simulink model "kopter_se_zavazim_Cascade_PID"  (R2024b)
settings: Solver=ode4  StartTime=0.0  StopTime=16  FixedStep=0.01  RelTol=1e-3
values from neighbouring files (symbols this model uses):
  A = 0.6081    [parametry_kopter_se_zavazim.m]
  b_moment = 3.6e-7    (= 3.6e-07)    [parametry_kopter_se_zavazim.m]
  d = 1    [parametry_kopter_se_zavazim.m]
  g = 9.81    [parametry_kopter_se_zavazim.m]
  Ip = m*d^2    (= 1)    [parametry_kopter_se_zavazim.m]
  Ixx = 0.0222    [parametry_kopter_se_zavazim.m]
  Iyy = 0.0222    [parametry_kopter_se_zavazim.m]
  Izz = 0.0429    [parametry_kopter_se_zavazim.m]
  k_thrust = 9.3e-6    (= 9.3e-06)    [parametry_kopter_se_zavazim.m]
  l = 0.2051    [parametry_kopter_se_zavazim.m]
  M = 2    [parametry_kopter_se_zavazim.m]
  m = 1    [parametry_kopter_se_zavazim.m]
  T = 0.8682    [parametry_kopter_se_zavazim.m]
  Us = [(M+m)*g; 0; 0; 0]    [parametry_kopter_se_zavazim.m]
  Xinit_ss = [Xinit_matrix; [0 0 0 0 0 0 0 0]']    [parametry_kopter_se_zavazim.m]
  Xs = [0;0;0; 0;0;0; 0;0; 0;0;0; 0;0;0; 0;0]    [parametry_kopter_se_zavazim.m]
undefined symbols (not defined in the file or in its folder): L, Us_p, Xs_p
libraries: simulink_extras x21, slpidlib x21, simulink x6
(part 5 of 5)

== matlab function kopter_se_zavazim_Cascade_PID/Nelinearni State-Space/B ==
  data: roll input; B output; pitch input; yaw input; alpha input; beta input; M parameter; Ixx parameter; Iyy parameter; Izz parameter; Ip parameter; d parameter; m parameter
function B = fcn(roll, pitch, yaw, alpha, beta, M, Ixx, Iyy, Izz, Ip, d, m)
% Matice vstupu do soustavy kvadrokoptery se zavazim

phi_t = roll;
theta_t = pitch;
psi_t = yaw;

alpha_t = alpha;
beta_t = beta;

B = [ 
                                                                                                                                                                                                                                                                                                                                                                                                                                                                                                                                                                                   0,                                                                                                                                                                           0,                                                                        0,                                                                                          0;
                                                                                                                                                                                                                                                                                                                                                                                                                                                                                                                                                                                   0,                                                                                                                                                                           0,                                                                        0,                                                                                          0;
                                                                                                                                                                                                                                                                                                                                                                                                                                                                                                                                                                                   0,                                                                                                                                                                           0,                                                                        0,                                                                                          0;
                                                                                                                                                                                                                                                                                                                                                                                                                                                                                                                                                                                   0,                                                                                                                                                                           0,                                                                        0,                                                                                          0;
                                                                                                                                                                                                                                                                                                                                                                                                                                                                                                                                                                                   0,                                                                                                                                                                           0,                                                                        0,                                                                                          0;
                                                                                                                                                                                                                                                                                                                                                                                                                                                                                                                                                                                   0,                                                                                                                                                                           0,                                                                        0,                                                                                          0;
                                                                                                                                                                                                                                                                                                                                                                                                                                                                                                                                                                                   0,                                                                                                                                                                           0,                                                                        0,                                                                                          0;
                                                                                                                                                                                                                                                                                                                                                                                                                                                                                                                                                                                   0,                                                                                                                                                                           0,                                                                        0,                                                                                          0;
(M*sin(phi_t)*sin(psi_t) + m*sin(phi_t)*sin(psi_t) + M*cos(phi_t)*cos(psi_t)*sin(theta_t) + m*cos(phi_t)*cos(psi_t)*sin(theta_t) - m*cos(beta_t)^2*sin(phi_t)*sin(psi_t) - m*cos(beta_t)^2*cos(phi_t)*cos(psi_t)*sin(theta_t) + m*cos(alpha_t)^2*cos(beta_t)^2*sin(phi_t)*sin(psi_t) + m*cos(alpha_t)*cos(beta_t)^2*cos(phi_t)*sin(alpha_t)*cos(theta_t) + m*cos(alpha_t)^2*cos(beta_t)^2*cos(phi_t)*cos(psi_t)*sin(theta_t) + m*cos(beta_t)*cos(psi_t)*sin(alpha_t)*sin(beta_t)*sin(phi_t) - m*cos(beta_t)*cos(phi_t)*sin(alpha_t)*sin(beta_t)*sin(psi_t)*sin(theta_t))/(M*(M + m)),                                                                                                                                                                           0,                                                                        0,                                                                                          0;
                                                                                                                                                                                              -(M*cos(psi_t)*sin(phi_t) - M*cos(phi_t)*sin(psi_t)*sin(theta_t) + m*cos(beta_t)^2*cos(psi_t)*sin(phi_t) - m*cos(beta_t)^2*cos(phi_t)*sin(psi_t)*sin(theta_t) + m*cos(beta_t)*sin(alpha_t)*sin(beta_t)*sin(phi_t)*sin(psi_t) - m*cos(alpha_t)*cos(beta_t)*cos(phi_t)*sin(beta_t)*cos(theta_t) + m*cos(beta_t)*cos(phi_t)*cos(psi_t)*sin(alpha_t)*sin(beta_t)*sin(theta_t))/(M*(M + m)),                                                                                                                                                                           0,                                                                        0,                                                                                          0;
                                                                                                                                                            (M*cos(phi_t)*cos(theta_t) + m*cos(phi_t)*cos(theta_t) - m*cos(alpha_t)^2*cos(beta_t)^2*cos(phi_t)*cos(theta_t) + m*cos(alpha_t)*cos(beta_t)^2*sin(alpha_t)*sin(phi_t)*sin(psi_t) - m*cos(alpha_t)*cos(beta_t)*cos(psi_t)*sin(beta_t)*sin(phi_t) + m*cos(alpha_t)*cos(beta_t)^2*cos(phi_t)*cos(psi_t)*sin(alpha_t)*sin(theta_t) + m*cos(alpha_t)*cos(beta_t)*cos(phi_t)*sin(beta_t)*sin(psi_t)*sin(theta_t))/(M*(M + m)),                                                                                                                                                                           0,                                                                        0,                                                                                          0;
                                                                                                                                                                                                                                                                                                                                                                                                                                                                                                                                                                                   0, -(Iyy*Izz + Ixx*Iyy*sin(theta_t)^2 - Iyy*Izz*sin(theta_t)^2 - Ixx*Iyy*sin(phi_t)^2*sin(theta_t)^2 + Ixx*Izz*sin(phi_t)^2*sin(theta_t)^2)/(Ixx*Iyy*Izz*(sin(theta_t)^2 - 1)), -(cos(phi_t)*sin(phi_t)*sin(theta_t)*(Iyy - Izz))/(Iyy*Izz*cos(theta_t)), -(sin(theta_t)*(Iyy - Iyy*sin(phi_t)^2 + Izz*sin(phi_t)^2))/(Iyy*Izz*(sin(theta_t)^2 - 1));
                                                                                                                                                                                                                                                                                                                                                                                                                                                                                                                                                                                   0,                                                                                                    -(cos(phi_t)*sin(phi_t)*sin(theta_t)*(Iyy - Izz))/(Iyy*Izz*cos(theta_t)),                    (Izz + Iyy*sin(phi_t)^2 - Izz*sin(phi_t)^2)/(Iyy*Izz),                                       -(sin(2*phi_t)*(Iyy - Izz))/(2*Iyy*Izz*cos(theta_t));
                                                                                                                                                                                                                                                                                                                                                                                                                                                                                                                                                                                   0,                                                                                  -(sin(theta_t)*(Iyy - Iyy*sin(phi_t)^2 + Izz*sin(phi_t)^2))/(Iyy*Izz*(sin(theta_t)^2 - 1)),                     -(sin(2*phi_t)*(Iyy - Izz))/(2*Iyy*Izz*cos(theta_t)),                -(Iyy - Iyy*sin(phi_t)^2 + Izz*sin(phi_t)^2)/(Iyy*Izz*(sin(theta_t)^2 - 1));
                                                                                                                                                                                                                                                                                                                                                                                                                                    -(cos(phi_t)*sin(alpha_t)*cos(theta_t) + cos(alpha_t)*sin(phi_t)*sin(psi_t) + cos(alpha_t)*cos(phi_t)*cos(psi_t)*sin(theta_t))/(M*d*cos(beta_t)),                                                                                                                                                                           0,                                                                        0,                                                                                          0;
                                                                                                                                                                                                                                                                                                                        (cos(beta_t)*cos(psi_t)*sin(phi_t) - cos(alpha_t)*cos(phi_t)*sin(beta_t)*cos(theta_t) - cos(beta_t)*cos(phi_t)*sin(psi_t)*sin(theta_t) + sin(alpha_t)*sin(beta_t)*sin(phi_t)*sin(psi_t) + cos(phi_t)*cos(psi_t)*sin(alpha_t)*sin(beta_t)*sin(theta_t))/(M*d),                                                                                                                                                                           0,                                                                        0,                                                                                          0];

== matlab function kopter_se_zavazim_Cascade_PID/Nelinearni State-Space/BQ ==
  data: BQ output; g parameter
function BQ = fcn(g)
% Matice vstupu tihy
BQ = [0 0 0 0 0 0 0 0 0 0 -g 0 0 0 0 0]';

== matlab function kopter_se_zavazim_Cascade_PID/Nelinearni State-Space/MATLAB Function ==
  data: u output; m1 input; m2 input; m3 input; m4 input; k_thrust parameter; b_moment parameter; L parameter
function u = fcn(m1, m2, m3, m4, k_thrust, b_moment, L)

Thrust = k_thrust*(m1^2 + m2^2 + m3^2 + m4^2);
Tau_roll = L*k_thrust*(m1^2 + m4^2 - m2^2 - m3^2);
Tau_pitch = L*k_thrust*(m4^2 + m3^2 - m1^2 - m2^2);
Tau_yaw = b_moment*(m1^2 + m3^2 - m2^2 - m4^2);

u = [Thrust; Tau_roll; Tau_pitch; Tau_yaw];

== matlab function kopter_se_zavazim_Cascade_PID/Linearni State-Space__/MATLAB Function ==
  data: u output; m1 input; m2 input; m3 input; m4 input; k_thrust parameter; b_moment parameter; l parameter
function u = fcn(m1, m2, m3, m4, k_thrust, b_moment, l)

Thrust = k_thrust*(m1^2 + m2^2 + m3^2 + m4^2);
Tau_roll = l*k_thrust*(m1^2 + m4^2 - m2^2 - m3^2);
Tau_pitch = l*k_thrust*(m4^2 + m3^2 - m1^2 - m2^2);
Tau_yaw = b_moment*(m1^2 + m3^2 - m2^2 - m4^2);

u = [Thrust; Tau_roll; Tau_pitch; Tau_yaw];

== matlab function kopter_se_zavazim_Cascade_PID/Linearni State-Space_/Ac ==
  data: g parameter; M parameter; Ac output; m parameter; d parameter
function Ac = fcn(g, M, m, d)
% Matice Ac linearizovana kvadrokoptera+zavazi

Ac = [
0, 0, 0,                 0,                  0, 0,                  0,                  0, 1, 0, 0, 0, 0, 0, 0, 0;
0, 0, 0,                 0,                  0, 0,                  0,                  0, 0, 1, 0, 0, 0, 0, 0, 0;
0, 0, 0,                 0,                  0, 0,                  0,                  0, 0, 0, 1, 0, 0, 0, 0, 0;
0, 0, 0,                 0,                  0, 0,                  0,                  0, 0, 0, 0, 1, 0, 0, 0, 0;
0, 0, 0,                 0,                  0, 0,                  0,                  0, 0, 0, 0, 0, 1, 0, 0, 0;
0, 0, 0,                 0,                  0, 0,                  0,                  0, 0, 0, 0, 0, 0, 1, 0, 0;
0, 0, 0,                 0,                  0, 0,                  0,                  0, 0, 0, 0, 0, 0, 0, 1, 0;
0, 0, 0,                 0,                  0, 0,                  0,                  0, 0, 0, 0, 0, 0, 0, 0, 1;
0, 0, 0,                 0,      (g*(M + m))/M, 0,            (g*m)/M,                  0, 0, 0, 0, 0, 0, 0, 0, 0;
0, 0, 0,    -(g*(M + m))/M,                  0, 0,                  0,            (g*m)/M, 0, 0, 0, 0, 0, 0, 0, 0;
0, 0, 0,                 0,                  0, 0,                  0,                  0, 0, 0, 0, 0, 0, 0, 0, 0;
0, 0, 0,                 0,                  0, 0,                  0,                  0, 0, 0, 0, 0, 0, 0, 0, 0;
0, 0, 0,                 0,                  0, 0,                  0,                  0, 0, 0, 0, 0, 0, 0, 0, 0;
0, 0, 0,                 0,                  0, 0,                  0,                  0, 0, 0, 0, 0, 0, 0, 0, 0;
0, 0, 0,                 0, -(g*(M + m))/(M*d), 0, -(g*(M + m))/(M*d),                  0, 0, 0, 0, 0, 0, 0, 0, 0;
0, 0, 0, (g*(M + m))/(M*d),                  0, 0,                  0, -(g*(M + m))/(M*d), 0, 0, 0, 0, 0, 0, 0, 0];

== matlab function kopter_se_zavazim_Cascade_PID/MATLAB Function1 ==
  data: x_ref output; y_ref output; z_ref output; sim_time input; yaw_ref output
function [x_ref, y_ref, z_ref, yaw_ref] = fcn(sim_time)
if sim_time < 10
    z_ref = 8;
    x_ref = 0;
    y_ref = 0;
    yaw_ref = 0;
elseif sim_time < 20
    z_ref = 15;
    x_ref = 10;
    y_ref = 0;
    yaw_ref = 45;
elseif sim_time < 25
    z_ref = 8;
    x_ref = 10;
    y_ref = -5;
    yaw_ref = -45;
elseif sim_time < 30
    z_ref = 10;
    x_ref = -5;
    y_ref = -10;
    yaw_ref = -15;
elseif sim_time < 40
    z_ref = 12;
    x_ref = -5;
    y_ref = 0;
    yaw_ref = 30;
else
    x_ref = 0; % [m]
    y_ref = 0; % [m]
    z_ref = 10; % [m]
    yaw_ref = 0; %[deg] mezi -180 deg a +180 deg
end

== matlab function kopter_se_zavazim_Cascade_PID/Motors command calculation ==
  data: thrust_cmd input; U1 output; roll_cmd input; pitch_cmd input; yaw_cmd input; U2 output; U3 output; U4 output
function [U1, U2, U3, U4] = fcn(thrust_cmd, roll_cmd, pitch_cmd, yaw_cmd)

U1 = thrust_cmd+roll_cmd-pitch_cmd+yaw_cmd;
U2 = thrust_cmd-roll_cmd-pitch_cmd-yaw_cmd;
U3 = thrust_cmd-roll_cmd+pitch_cmd+yaw_cmd;
U4 = thrust_cmd+roll_cmd+pitch_cmd-yaw_cmd;

== matlab function kopter_se_zavazim_Cascade_PID/World to Body ==
  data: x_ref input; x_ref_ output; y_ref input; yaw input; y_ref_ output
function [x_ref_, y_ref_]= fcn(x_ref, y_ref, yaw)
R_z = [cos(yaw), -sin(yaw), 0; 
       sin(yaw), cos(yaw), 0; 
       0, 0, 1];

out = R_z\[x_ref; y_ref; 0];
%out = [x_ref, y_ref];
x_ref_ = out(1);
y_ref_ = out(2);
